simulink model "Driveline"  (R2018a)
settings: Solver=ode23tb  StartTime=0.0  StopTime=inf  FixedStep=.001  RelTol=1e-3
model workspace (MAT data in the model file):
  Trans.InputShaftInertia = 0.01
  Trans.InputShaftDamping = 0.001
  Trans.FinalDrive = 2.77
  Trans.GearRatios = [-3.82 4.56 4.56 2.97 2.08 1.69 1.27 1 0.85 0.65]
  Trans.GearNums = [-1 0 1 2 3 4 5 6 7 8]
  Trans.Inertias = [0.128 0.128 0.128 0.1 0.062 0.028 0.01 0.01 0.01 0.01]
  Trans.DampingCoeffs = [0.003 0.001 0.003 0.0025 0.002 0.001 0.001 0.001 0.001 0.001]
  Trans.Efficiencies = [0.9 0.9 0.9 0.9 0.9 0.95 0.95 0.95 0.95 0.95]
  Trans.ShiftTau = 0.02
libraries: autolibsharedcoupling x9, autolibshareddiff x4, autolibutils x1, vehdynlibsteering x1, autolibsharedtransfixedgear x1
settings Model: ModifiedByFormat=The MathWorks, Inc.  Creator=The MathWorks, Inc.  LastModifiedBy=The MathWorks, Inc.
settings SolverCC: ZeroCrossControl=DisableAll  DecoupledContinuousIntegration=on
settings DebuggingCC: ArtificialAlgebraicLoopMsg=none  IgnoredZcDiagnostic=none
settings ModelReferenceCC: ModelReferenceMinAlgLoopOccurrences=on

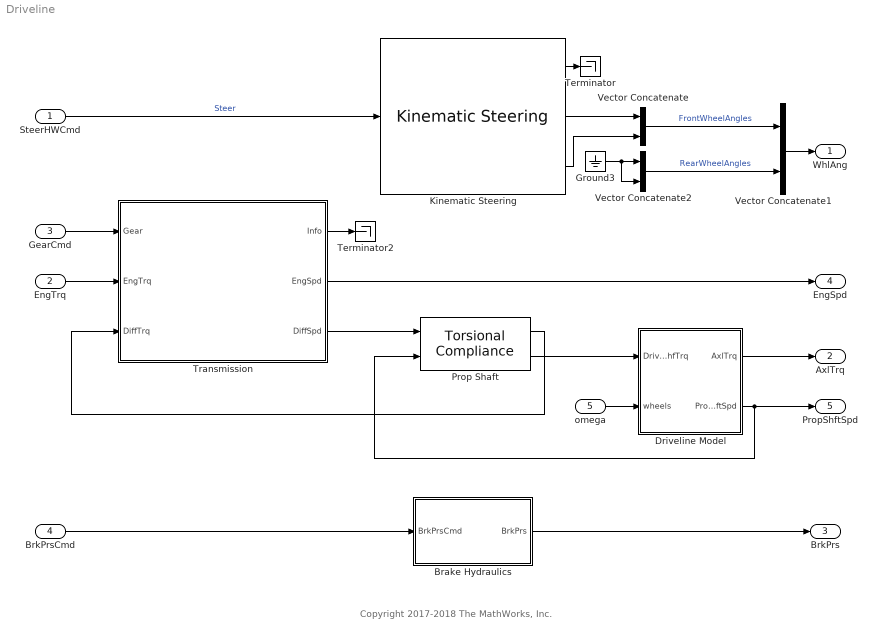
== system Driveline ==
  note: Copyright 2017-2018 The MathWorks, Inc.
  SteerHWCmd : Inport
  EngTrq : Inport  Port=2
  GearCmd : Inport  Port=3  OutDataTypeStr=int8
  BrkPrsCmd : Inport  Port=4  PortDimensions=4
  omega : Inport  Port=5
  Brake Hydraulics : Subsystem
  Driveline Model : Subsystem  Variant=on  OverrideUsingVariant=0
  Ground3 : Ground
  Kinematic Steering : vehdynlibsteering/Kinematic Steering  StrgType=Ackerman  StrgRatioType=Constant  Loc=Front  NrmlFctr=1  TrckWdth=1.922  WhlBase=(1.515+1.504)  Db=0  StrgRng=3*pi  StrgAngBpts="[-6.2832   -5.0265   -3.7699   -2.5133   -1.2566         0    1.2566    2.5133    3.7699    5.0265    6.2832]"  StrgRatioTbl=|  StrgRatio=18  StrgArmLngth=0.1  RckCsLngth=0.5  TieRodLngth=0.248128028933392  D=0.2  PnnRadius=0.0057  PnnRadiusTbl="[0.0055    0.0055    0.0056    0.0057    0.0057    0.0057    0.0057    0.0057    0.0056    0.0055    0.0055]"  RodLngth=0.1  ParaArmLngth=0.9  aMode=2
      | [13.5000   13.3750   13.2500   13.1250   13.0000   13.0000   13.0000   13.1250   13.2500   13.3750   13.5000
      | ]
      settings: SourceProductName=Vehicle Dynamics Blockset
  Prop Shaft : autolibsharedcoupling/Torsional Compliance  port_config=Simulink  k=5e3  b=50  theta_o=0  domega_o=0  omega_c=150  blkID=0  aMode=2
      settings: SourceProductName=Powertrain Blockset  SourceProductBaseCode=PW
  Terminator : Terminator
  Terminator2 : Terminator
  Transmission : Subsystem  Variant=on  OverrideUsingVariant=0
  Vector Concatenate : Concatenate
  Vector Concatenate1 : Concatenate
  Vector Concatenate2 : Concatenate
  WhlAng : Outport  Unit=rad
  AxlTrq : Outport  Port=2
  BrkPrs : Outport  Port=3  PortDimensions=4
  EngSpd : Outport  Port=4  Unit=rad/s
  PropShftSpd : Outport  Port=5
  wires:
  Vector Concatenate1/1 -> WhlAng/1
  Vector Concatenate2/1 -> Vector Concatenate1/2  "RearWheelAngles"
  Transmission/2(EngSpd) -> EngSpd/1
  SteerHWCmd/1 -> Kinematic Steering/1  "Steer"
  Ground3/1 -> Vector Concatenate2/2, Vector Concatenate2/1
  GearCmd/1 -> Transmission/1(Gear)
  Kinematic Steering/1 -> Terminator/1
  Kinematic Steering/3 -> Vector Concatenate/2
  BrkPrsCmd/1 -> Brake Hydraulics/1(BrkPrsCmd)
  Kinematic Steering/2 -> Vector Concatenate/1
  Prop Shaft/2 -> Driveline Model/1(DriveshfTrq)
  EngTrq/1 -> Transmission/2(EngTrq)
  Transmission/1(Info) -> Terminator2/1
  Vector Concatenate/1 -> Vector Concatenate1/1  "FrontWheelAngles"
  Prop Shaft/1 -> Transmission/3(DiffTrq)
  Driveline Model/2(PropShaftSpd) -> Prop Shaft/2, PropShftSpd/1
  omega/1 -> Driveline Model/2(wheels)
  Brake Hydraulics/1(BrkPrs) -> BrkPrs/1
  Transmission/3(DiffSpd) -> Prop Shaft/1
  Driveline Model/1(AxlTrq) -> AxlTrq/1

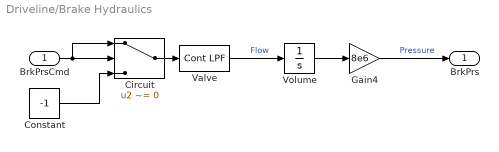
== system Driveline/Brake Hydraulics ==
  BrkPrsCmd : Inport
  Circuit : Switch  Criteria=u2 ~= 0
  Constant : Constant  Value=-1
  Gain4 : Gain  Gain=8e6
  Valve : autolibutils/Cont LPF  wc=200*2*pi  aMode=2
      settings: SourceProductName=Powertrain Blockset  SourceProductBaseCode=PW
  Volume : Integrator  LimitOutput=on  UpperSaturationLimit=1  LowerSaturationLimit=0
  BrkPrs : Outport
  wires:
  Volume/1 -> Gain4/1
  Valve/1 -> Volume/1  "Flow"
  BrkPrsCmd/1 -> Circuit/1, Circuit/2
  Gain4/1 -> BrkPrs/1  "Pressure"
  Circuit/1 -> Valve/1
  Constant/1 -> Circuit/3

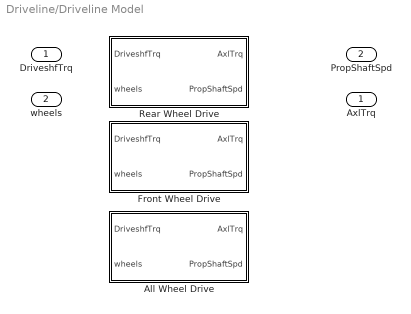
== system Driveline/Driveline Model ==
  DriveshfTrq : Inport
  wheels : Inport  Port=2
  All Wheel Drive : Subsystem  VariantControl=2
  Front Wheel Drive : Subsystem  VariantControl=1
  Rear Wheel Drive : Subsystem  VariantControl=0
  AxlTrq : Outport
  PropShaftSpd : Outport  Port=2

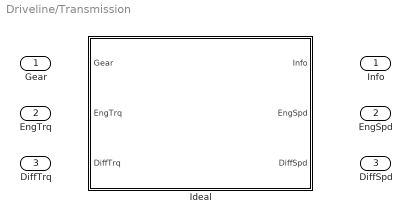
== system Driveline/Transmission ==
  Gear : Inport
  EngTrq : Inport  Port=2
  DiffTrq : Inport  Port=3
  Ideal : Subsystem  VariantControl=0
  Info : Outport
  EngSpd : Outport  Port=2
  DiffSpd : Outport  Port=3

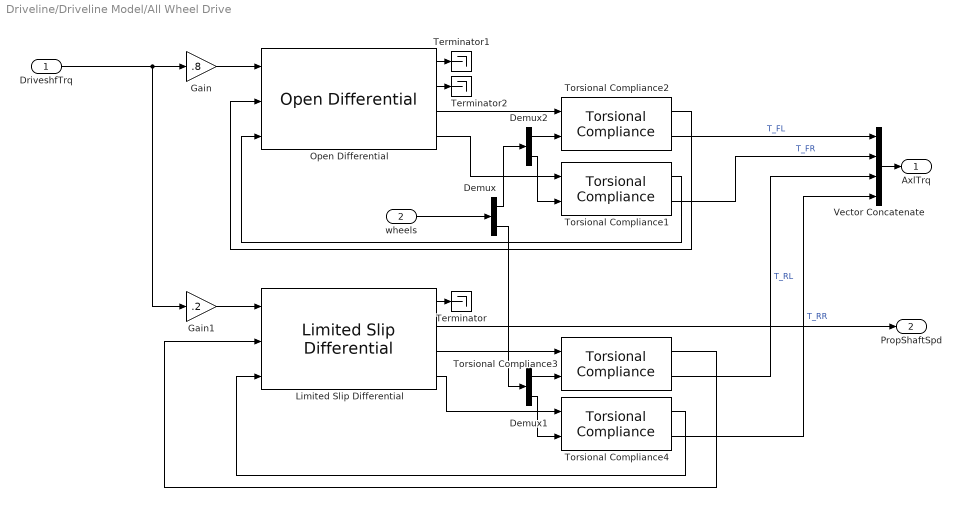
== system Driveline/Driveline Model/All Wheel Drive ==
  DriveshfTrq : Inport
  wheels : Inport  Port=2
  Demux : Demux  Outputs=[2,2]
  Demux1 : Demux  Outputs=2
  Demux2 : Demux  Outputs=2
  Gain : Gain  Gain=.8
  Gain1 : Gain  Gain=.2
  Limited Slip Differential : autolibshareddiff/Limited Slip Differential  shaftSwitchMask=To the left of center-line  Ndiff=Trans.FinalDrive  Jd=.08  bd=1e-3  Jw1=.05  bw1=1e-3  Jw2=.05  bw2=1e-3  omegaw1o=0  omegaw2o=0  couplingType=Pre-loaded ideal clutch  Ndisks=8  Reff=.08  Fc=1000  muc=[.16 0.13 0.115 0.11 0.105 0.1025 0.10125 .10125]  dw=[0 10 20 40 60 80 100 1000]  Tdw=[-100, -90, -50, -5, 0, 5, 50, 90, 100]  dwT=[-200, -175, -100, - 50, 0, 50, 100, 175, 200]  TTin=[-200 -175 -100 - 50 0 50 100 175 200]  Tin=[-200 -175 -100 - 50 0 50 100 175 200]  tauC=.04  IdealInterpMethod=Linear  IdealExtrapMethod=Linear  TdwInterpMethod=Flat  TdwExtrapMethod=Clip  TTinInterpMethod=Flat  TTinExtrapMethod=Clip  maxAbsSpd=5e3  aMode=2
      settings: SourceProductName=Powertrain Blockset  SourceProductBaseCode=PW
  Open Differential : autolibshareddiff/Open Differential  shaftSwitchMask=To the left of center-line  Ndiff=4.5  Jd=.1  bd=1e-3  Jw1=.1  bw1=1e-3  Jw2=.1  bw2=1e-3  omegaw1o=0  omegaw2o=0  maxAbsSpd=5e3  aMode=2
      settings: SourceProductName=Powertrain Blockset  SourceProductBaseCode=PW
  Terminator : Terminator
  Terminator1 : Terminator
  Terminator2 : Terminator
  Torsional Compliance{1..4} (4 alike) : autolibsharedcoupling/Torsional Compliance  port_config=Simulink  k=3e5  b=50  theta_o=0  domega_o=0  omega_c=150  blkID=0  aMode=2
      settings: SourceProductName=Powertrain Blockset  SourceProductBaseCode=PW
  Vector Concatenate : Concatenate  NumInputs=4
  AxlTrq : Outport
  PropShaftSpd : Outport  Port=2
  wires:
  Torsional Compliance3/1 -> Limited Slip Differential/2
  Torsional Compliance4/1 -> Limited Slip Differential/3
  Demux/2 -> Demux1/1
  Demux1/2 -> Torsional Compliance4/2
  Limited Slip Differential/4 -> Torsional Compliance4/1
  Limited Slip Differential/1 -> Terminator/1
  Demux1/1 -> Torsional Compliance3/2
  Limited Slip Differential/3 -> Torsional Compliance3/1
  Demux/1 -> Demux2/1
  wheels/1 -> Demux/1
  DriveshfTrq/1 -> Gain1/1, Gain/1
  Open Differential/3 -> Torsional Compliance2/1
  Open Differential/4 -> Torsional Compliance1/1
  Demux2/1 -> Torsional Compliance2/2
  Demux2/2 -> Torsional Compliance1/2
  Torsional Compliance1/1 -> Open Differential/3
  Torsional Compliance2/1 -> Open Differential/2
  Limited Slip Differential/2 -> PropShaftSpd/1
  Open Differential/1 -> Terminator1/1
  Open Differential/2 -> Terminator2/1
  Gain/1 -> Open Differential/1
  Gain1/1 -> Limited Slip Differential/1
  Torsional Compliance4/2 -> Vector Concatenate/4  "T_RR"
  Torsional Compliance1/2 -> Vector Concatenate/2  "T_FR"
  Torsional Compliance3/2 -> Vector Concatenate/3  "T_RL"
  Torsional Compliance2/2 -> Vector Concatenate/1  "T_FL"
  Vector Concatenate/1 -> AxlTrq/1

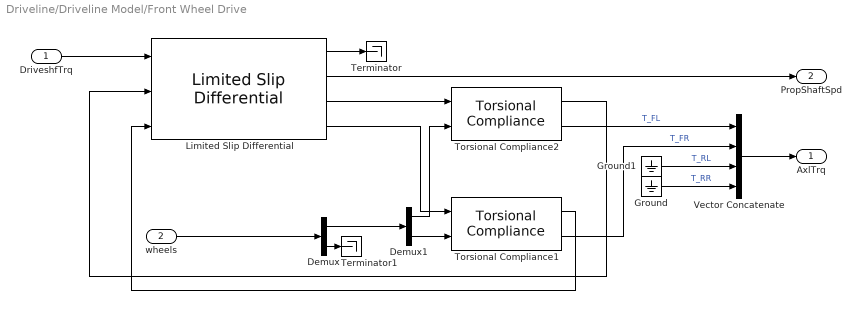
== system Driveline/Driveline Model/Front Wheel Drive ==
  DriveshfTrq : Inport
  wheels : Inport  Port=2
  Demux : Demux  Outputs=[2,2]
  Demux1 : Demux  Outputs=2
  Ground : Ground
  Ground1 : Ground
  Limited Slip Differential : autolibshareddiff/Limited Slip Differential  shaftSwitchMask=To the left of center-line  Ndiff=Trans.FinalDrive  Jd=.08  bd=1e-3  Jw1=.05  bw1=1e-3  Jw2=.05  bw2=1e-3  omegaw1o=0  omegaw2o=0  couplingType=Pre-loaded ideal clutch  Ndisks=8  Reff=.08  Fc=1000  muc=[.16 0.13 0.115 0.11 0.105 0.1025 0.10125 .10125]  dw=[0 10 20 40 60 80 100 1000]  Tdw=[-100, -90, -50, -5, 0, 5, 50, 90, 100]  dwT=[-200, -175, -100, - 50, 0, 50, 100, 175, 200]  TTin=[-200 -175 -100 - 50 0 50 100 175 200]  Tin=[-200 -175 -100 - 50 0 50 100 175 200]  tauC=.04  IdealInterpMethod=Linear  IdealExtrapMethod=Linear  TdwInterpMethod=Flat  TdwExtrapMethod=Clip  TTinInterpMethod=Flat  TTinExtrapMethod=Clip  maxAbsSpd=5e3  aMode=2
      settings: SourceProductName=Powertrain Blockset  SourceProductBaseCode=PW
  Terminator : Terminator
  Terminator1 : Terminator
  Torsional Compliance1 : autolibsharedcoupling/Torsional Compliance  port_config=Simulink  k=3e5  b=50  theta_o=0  domega_o=0  omega_c=150  blkID=0  aMode=2
      settings: SourceProductName=Powertrain Blockset  SourceProductBaseCode=PW
  Torsional Compliance2 : autolibsharedcoupling/Torsional Compliance  port_config=Simulink  k=3e5  b=50  theta_o=0  domega_o=0  omega_c=150  blkID=0  aMode=2
      settings: SourceProductName=Powertrain Blockset  SourceProductBaseCode=PW
  Vector Concatenate : Concatenate  NumInputs=4
  AxlTrq : Outport
  PropShaftSpd : Outport  Port=2
  wires:
  Limited Slip Differential/3 -> Torsional Compliance2/1
  Demux1/1 -> Torsional Compliance2/2
  Limited Slip Differential/1 -> Terminator/1
  DriveshfTrq/1 -> Limited Slip Differential/1
  Limited Slip Differential/2 -> PropShaftSpd/1
  Limited Slip Differential/4 -> Torsional Compliance1/1
  Demux1/2 -> Torsional Compliance1/2
  Demux/1 -> Demux1/1
  Torsional Compliance1/1 -> Limited Slip Differential/3
  Torsional Compliance2/1 -> Limited Slip Differential/2
  Demux/2 -> Terminator1/1
  Ground/1 -> Vector Concatenate/4  "T_RR"
  Torsional Compliance1/2 -> Vector Concatenate/2  "T_FR"
  Ground1/1 -> Vector Concatenate/3  "T_RL"
  Torsional Compliance2/2 -> Vector Concatenate/1  "T_FL"
  wheels/1 -> Demux/1
  Vector Concatenate/1 -> AxlTrq/1

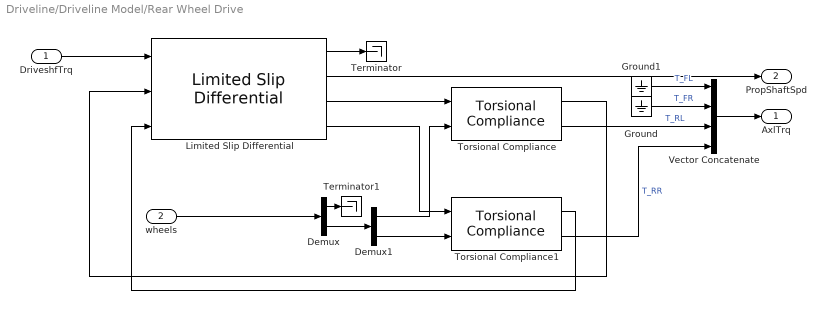
== system Driveline/Driveline Model/Rear Wheel Drive ==
  DriveshfTrq : Inport
  wheels : Inport  Port=2
  Demux : Demux  Outputs=[2,2]
  Demux1 : Demux  Outputs=2
  Ground : Ground
  Ground1 : Ground
  Limited Slip Differential : autolibshareddiff/Limited Slip Differential  shaftSwitchMask=To the left of center-line  Ndiff=Trans.FinalDrive  Jd=.08  bd=1e-3  Jw1=.01  bw1=1e-3  Jw2=.01  bw2=1e-3  omegaw1o=0  omegaw2o=0  couplingType=Pre-loaded ideal clutch  Ndisks=8  Reff=.08  Fc=1000  muc=[.16 0.13 0.115 0.11 0.105 0.1025 0.10125 .10125]  dw=[0 10 20 40 60 80 100 1000]  Tdw=[-100, -90, -50, -5, 0, 5, 50, 90, 100]  dwT=[-200, -175, -100, - 50, 0, 50, 100, 175, 200]  TTin=[-200 -175 -100 - 50 0 50 100 175 200]  Tin=[-200 -175 -100 - 50 0 50 100 175 200]  tauC=.04  IdealInterpMethod=Linear  IdealExtrapMethod=Linear  TdwInterpMethod=Flat  TdwExtrapMethod=Clip  TTinInterpMethod=Flat  TTinExtrapMethod=Clip  maxAbsSpd=5e3  aMode=2
      settings: SourceProductName=Powertrain Blockset  SourceProductBaseCode=PW
  Terminator : Terminator
  Terminator1 : Terminator
  Torsional Compliance : autolibsharedcoupling/Torsional Compliance  port_config=Simulink  k=5e3  b=50  theta_o=0  domega_o=0  omega_c=150  blkID=0  aMode=2
      settings: SourceProductName=Powertrain Blockset  SourceProductBaseCode=PW
  Torsional Compliance1 : autolibsharedcoupling/Torsional Compliance  port_config=Simulink  k=5e3  b=50  theta_o=0  domega_o=0  omega_c=150  blkID=0  aMode=2
      settings: SourceProductName=Powertrain Blockset  SourceProductBaseCode=PW
  Vector Concatenate : Concatenate  NumInputs=4
  AxlTrq : Outport
  PropShaftSpd : Outport  Port=2
  wires:
  Torsional Compliance/1 -> Limited Slip Differential/2
  Torsional Compliance1/1 -> Limited Slip Differential/3
  Demux/2 -> Demux1/1
  Demux1/2 -> Torsional Compliance1/2
  Limited Slip Differential/4 -> Torsional Compliance1/1
  Limited Slip Differential/2 -> PropShaftSpd/1
  DriveshfTrq/1 -> Limited Slip Differential/1
  Limited Slip Differential/1 -> Terminator/1
  Demux1/1 -> Torsional Compliance/2
  Limited Slip Differential/3 -> Torsional Compliance/1
  Demux/1 -> Terminator1/1
  wheels/1 -> Demux/1
  Torsional Compliance1/2 -> Vector Concatenate/4  "T_RR"
  Ground/1 -> Vector Concatenate/2  "T_FR"
  Ground1/1 -> Vector Concatenate/1  "T_FL"
  Torsional Compliance/2 -> Vector Concatenate/3  "T_RL"
  Vector Concatenate/1 -> AxlTrq/1

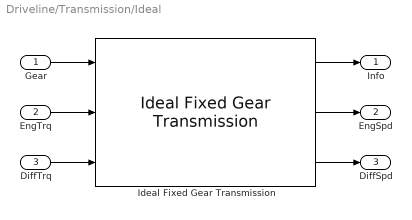
== system Driveline/Transmission/Ideal ==
  Gear : Inport
  EngTrq : Inport  Port=2
  DiffTrq : Inport  Port=3
  Ideal Fixed Gear Transmission : autolibsharedtransfixedgear/Ideal Fixed Gear Transmission  VariantControl=0  TransEffModelPopup=Gear only  gearInterp=Nearest  G=Trans.GearNums  Trq_bpts=[25, 50, 75, 100, 150, 200, 250]  omega_bpts=[52.4 78.5 105 131 157 183 209 262 314 419 524]  Temp_bpts=[313 358]  N=Trans.GearRatios  Jout=Trans.Inertias  bout=Trans.DampingCoeffs  eta=Trans.Efficiencies  eta_tbl=reshape([0.53 0.71 0.77 0.79 0.82 0.82 0.82 0.5 0.7 0.77 0.79 0.82 0.82 0.82 0.54 0.72 0.78 0.81 0.83 0.82 0.82 0.56 0.73 0.79 0.81 0.84 0.82 0.82 0.58 0.74 0.79 0.82 0.84 0.82 0.82 0.57 0.74 0.79 0.82 0.84 0.82 0.82 0.58 0.74 0.79 0.82 0.84 0.82 0.82 0.58 0.74 0.79 0.82 0.84 0.82 0.82 0.57 0.74 0.8 0.82 0.85 0.82 0.82 0.55 0.73 0.78 0.81 0.84 0.82 0.82 0.51 0.71 0.77 0.81 0.84 0.82 0.82 0.53 0.71 0.77 0.79 0.82 0.82 0.82 0.5 0.7 0.77 0.79 0.82 0.82 0.82 0.54 0.72 0.78 0.81 0.83 0.82 0.82 0.56 0.73 0.79 0.81 0.84 0.82 0.82 0.58 0.74 0.79 0.82 0.84 0.82 0.82 0.57 0.74 0.79 0.82 0.84 0.82 0.82 0.58 0.74 0.79 0.82 0.84 0.82 0.82 0.58 0.74 0.79 0.82 0.84 0.82 0.82 0.57 0.74 0.8 0.82 0.85 0.82 0.82 0.55 0.73 0.78 0.81 0.84 0.82 0.82 0.51 0.71 0.77 0.81 0.84 0.82 0.82 0.53 0.71 0.77 0.79 0.82 0.82 0.82 0.5 0.7 0.77 0.79 0.82 0.82 0.82 0.54 0.72 0.78 0.81 0.83 0.82 0.82 0.56 0.73 0.79 0.81 0.84 0.82 0.82 0.58 0.74 0.79 0.82 0.84 0.82 0.82 0.57 0.74 0.79 0.82 0.84 0.82 0.82 0.58 0.74 0.79 0.82 0.84 0.82 0.82 0.58 0.74 0.79 0.82 0.84 0.82 0.82 0.57 0.74 0.8 0.82 0.85 0.82 0.82 0.55 0.73 0.78 0.81 0.84 0.82 0.82 0.51 0.71 0.77 0.81 0.84 0.82 0.82 0.7 0.79 0.82 0.83 0.84 0.84 0.84 0.63 0.76 0.8 0.82 0.83 0.84 0.84 0.58 0.74 0.79 0.81 0.83 0.84 0.84 0.58 0.74 0.79 0.81 0.83 0.84 0.84 0.58 0.74 0.79 0.81 0.84 0.84 0.84 0.57 0.73 0.78 0.81 0.84 0.85 0.84 0.57 0.73 0.79 0.81 0.84 0.85 0.84 0.56 0.73 0.78 0.81 0.83 0.85 0.84 0.55 0.73 0.78 0.81 0.84 0.85 0.84 0.52 0.71 0.77 0.8 0.83 0.85 0.84 0.48 0.69 0.76 0.79 0.83 0.84 0.84 0.64 0.76 0.8 0.81 0.83 0.84 0.84 0.56 0.73 0.78 0.8 0.83 0.84 0.84 0.54 0.71 0.77 0.8 0.82 0.84 0.84 0.53 0.71 0.77 0.8 0.83 0.84 0.84 0.51 0.71 0.77 0.8 0.83 0.84 0.85 0.52 0.7 0.77 0.8 0.83 0.84 0.85 0.51 0.71 0.76 0.79 0.83 0.84 0.85 0.5 0.69 0.76 0.79 0.82 0.84 0.85 0.45 0.68 0.75 0.78 0.82 0.84 0.85 0.43 0.67 0.74 0.78 0.81 0.83 0.84 0.38 0.63 0.71 0.75 0.8 0.82 0.83 0.65 0.79 0.84 0.85 0.88 0.89 0.89 0.56 0.75 0.81 0.83 0.86 0.88 0.89 0.52 0.72 0.79 0.83 0.86 0.88 0.88 0.51 0.72 0.79 0.83 0.86 0.88 0.89 0.49 0.71 0.78 0.82 0.86 0.88 0.89 0.47 0.7 0.78 0.82 0.86 0.87 0.88 0.45 0.69 0.77 0.81 0.85 0.87 0.88 0.4 0.67 0.75 0.8 0.84 0.86 0.88 0.3 0.64 0.73 0.78 0.83 0.86 0.87 0.17 0.55 0.67 0.73 0.8 0.83 0.85 0.089 0.45 0.61 0.69 0.77 0.81 0.83 0.61 0.75 0.82 0.84 0.87 0.87 0.88 0.54 0.73 0.8 0.82 0.86 0.87 0.88 0.51 0.71 0.79 0.82 0.86 0.87 0.88 0.52 0.72 0.79 0.82 0.86 0.87 0.89 0.52 0.72 0.8 0.83 0.86 0.88 0.89 0.53 0.72 0.79 0.82 0.86 0.87 0.89 0.5 0.7 0.78 0.82 0.86 0.88 0.88 0.46 0.69 0.77 0.81 0.85 0.87 0.88 0.4 0.67 0.75 0.8 0.83 0.86 0.88 0.33 0.64 0.73 0.78 0.83 0.85 0.87 0.33 0.64 0.73 0.78 0.83 0.85 0.87 0.78 0.85 0.87 0.88 0.89 0.89 0.89 0.73 0.83 0.86 0.88 0.89 0.89 0.89 0.72 0.83 0.86 0.88 0.89 0.89 0.89 0.72 0.83 0.87 0.89 0.9 0.89 0.89 0.72 0.83 0.87 0.88 0.9 0.89 0.89 0.71 0.83 0.87 0.88 0.9 0.89 0.89 0.71 0.83 0.86 0.88 0.9 0.89 0.89 0.7 0.82 0.86 0.88 0.9 0.89 0.89 0.69 0.82 0.86 0.88 0.9 0.89 0.89 0.67 0.81 0.86 0.88 0.9 0.89 0.89 0.63 0.79 0.85 0.87 0.89 0.89 0.89 0.78 0.85 0.87 0.88 0.89 0.89 0.89 0.73 0.83 0.86 0.88 0.89 0.89 0.89 0.72 0.83 0.86 0.88 0.89 0.89 0.89 0.72 0.83 0.87 0.89 0.9 0.89 0.89 0.72 0.83 0.87 0.88 0.9 0.89 0.89 0.71 0.83 0.87 0.88 0.9 0.89 0.89 0.71 0.83 0.86 0.88 0.9 0.89 0.89 0.7 0.82 0.86 0.88 0.9 0.89 0.89 0.69 0.82 0.86 0.88 0.9 0.89 0.89 0.67 0.81 0.86 0.88 0.9 0.89 0.89 0.63 0.79 0.85 0.87 0.89 0.89 0.89 0.78 0.85 0.87 0.88 0.89 0.89 0.89 0.73 0.83 0.86 0.88 0.89 0.89 0.89 0.72 0.83 0.86 0.88 0.89 0.89 0.89 0.72 0.83 0.87 0.89 0.9 0.89 0.89 0.72 0.83 0.87 0.88 0.9 0.89 0.89 0.71 0.83 0.87 0.88 0.9 0.89 0.89 0.71 0.83 0.86 0.88 0.9 0.89 0.89 0.7 0.82 0.86 0.88 0.9 0.89 0.89 0.69 0.82 0.86 0.88 0.9 0.89 0.89 0.67 0.81 0.86 0.88 0.9 0.89 0.89 0.63 0.79 0.85 0.87 0.89 0.89 0.89 0.82 0.87 0.88 0.89 0.89 0.89 0.89 0.81 0.87 0.89 0.89 0.9 0.9 0.89 0.76 0.85 0.87 0.89 0.9 0.89 0.89 0.72 0.83 0.86 0.88 0.89 0.89 0.89 0.72 0.83 0.86 0.88 0.89 0.9 0.89 0.71 0.82 0.86 0.88 0.89 0.9 ...(+1314 chars))  omega_o=0  tau_s=Trans.ShiftTau  maxAbsSpd=5e3  aMode=2
      settings: SourceProductName=Powertrain Blockset  SourceProductBaseCode=PW
  Info : Outport
  EngSpd : Outport  Port=2
  DiffSpd : Outport  Port=3
  wires:
  EngTrq/1 -> Ideal Fixed Gear Transmission/2
  Ideal Fixed Gear Transmission/2 -> EngSpd/1
  Gear/1 -> Ideal Fixed Gear Transmission/1
  Ideal Fixed Gear Transmission/3 -> DiffSpd/1
  Ideal Fixed Gear Transmission/1 -> Info/1
  DiffTrq/1 -> Ideal Fixed Gear Transmission/3
